simulink model "LV_grid"  (R2021b)
settings: Solver=VariableStepAuto  StartTime=0  StopTime=5.0005  FixedStep=5e-4  RelTol=1e-3
model workspace (MAT data in the model file):
  P2_1 = 3450
  idx = 1
  time_counter = 1
libraries: spsGroundLib x97, spsStairGeneratorLib x96, spsPiSectionLineLib x90, spsThreePhasePISectionLineLib x90, spsVariableInductorLib x48, spsVariableResistorLib x48, spsRMSLib x36, spsThreePhaseVIMeasurementLib x34, spsACVoltageSourceLib x5, spsLinearTransformerLib x5, spsPower3phInstantaneousLib x1, spsThreePhaseMutualInductanceZ1Z0Lib x1
(part 6 of 6)

== system LV_grid/L8/L1 ==
  Pi Section Line : spsPiSectionLineLib/Pi Section Line  LConnTagsString=__new0  RConnTagsString=__new0  Phases=1  PiSections=1  Length=0.0025  Frequency=50  Resistance=0.274  Inductance=0.073  Capacitance=12.74e-9  Measurements=None  Measurements2=None
      settings: SourceProductBaseCode=PS
  Three-Phase PI Section Line : spsThreePhasePISectionLineLib/Three-Phase PI Section Line  LConnTagsString=a|b|c  RConnTagsString=A|B|C  Length=0.0025  Frequency=50  Resistances=[ 0.274 0.959]  Inductances=[ 0.073 0.079]  Capacitances=[12.74e-9 7.751e-9]
  A : PMIOPort  Side=Left
  B : PMIOPort  Port=2  Side=Left
  C : PMIOPort  Port=3  Side=Left
  N : PMIOPort  Port=4  Side=Left
  a : PMIOPort  Port=5  Side=Right
  b : PMIOPort  Port=6  Side=Right
  c : PMIOPort  Port=7  Side=Right
  n : PMIOPort  Port=8  Side=Right
  connections:
  Pi Section Line/LConn1 -- N/RConn1
  Pi Section Line/RConn1 -- n/RConn1
  C/RConn1 -- Three-Phase PI Section Line/LConn3
  B/RConn1 -- Three-Phase PI Section Line/LConn2
  A/RConn1 -- Three-Phase PI Section Line/LConn1
  Three-Phase PI Section Line/RConn3 -- c/RConn1
  Three-Phase PI Section Line/RConn2 -- b/RConn1
  Three-Phase PI Section Line/RConn1 -- a/RConn1

== system LV_grid/L8/L2 ==
  Pi Section Line : spsPiSectionLineLib/Pi Section Line  LConnTagsString=__new0  RConnTagsString=__new0  Phases=1  PiSections=1  Length=0.0025  Frequency=50  Resistance=0.274  Inductance=0.073  Capacitance=12.74e-9  Measurements=None  Measurements2=None
      settings: SourceProductBaseCode=PS
  Three-Phase PI Section Line : spsThreePhasePISectionLineLib/Three-Phase PI Section Line  LConnTagsString=a|b|c  RConnTagsString=A|B|C  Length=0.0025  Frequency=50  Resistances=[ 0.274 0.959]  Inductances=[ 0.073 0.079]  Capacitances=[12.74e-9 7.751e-9]
  A : PMIOPort  Side=Left
  B : PMIOPort  Port=2  Side=Left
  C : PMIOPort  Port=3  Side=Left
  N : PMIOPort  Port=4  Side=Left
  a : PMIOPort  Port=5  Side=Right
  b : PMIOPort  Port=6  Side=Right
  c : PMIOPort  Port=7  Side=Right
  n : PMIOPort  Port=8  Side=Right
  connections:
  Pi Section Line/LConn1 -- N/RConn1
  Pi Section Line/RConn1 -- n/RConn1
  C/RConn1 -- Three-Phase PI Section Line/LConn3
  B/RConn1 -- Three-Phase PI Section Line/LConn2
  A/RConn1 -- Three-Phase PI Section Line/LConn1
  Three-Phase PI Section Line/RConn3 -- c/RConn1
  Three-Phase PI Section Line/RConn2 -- b/RConn1
  Three-Phase PI Section Line/RConn1 -- a/RConn1

== system LV_grid/L8/L3 ==
  Pi Section Line : spsPiSectionLineLib/Pi Section Line  LConnTagsString=__new0  RConnTagsString=__new0  Phases=1  PiSections=1  Length=0.0025  Frequency=50  Resistance=0.274  Inductance=0.073  Capacitance=12.74e-9  Measurements=None  Measurements2=None
      settings: SourceProductBaseCode=PS
  Three-Phase PI Section Line : spsThreePhasePISectionLineLib/Three-Phase PI Section Line  LConnTagsString=a|b|c  RConnTagsString=A|B|C  Length=0.0025  Frequency=50  Resistances=[ 0.274 0.959]  Inductances=[ 0.073 0.079]  Capacitances=[12.74e-9 7.751e-9]
  A : PMIOPort  Side=Left
  B : PMIOPort  Port=2  Side=Left
  C : PMIOPort  Port=3  Side=Left
  N : PMIOPort  Port=4  Side=Left
  a : PMIOPort  Port=5  Side=Right
  b : PMIOPort  Port=6  Side=Right
  c : PMIOPort  Port=7  Side=Right
  n : PMIOPort  Port=8  Side=Right
  connections:
  Pi Section Line/LConn1 -- N/RConn1
  Pi Section Line/RConn1 -- n/RConn1
  C/RConn1 -- Three-Phase PI Section Line/LConn3
  B/RConn1 -- Three-Phase PI Section Line/LConn2
  A/RConn1 -- Three-Phase PI Section Line/LConn1
  Three-Phase PI Section Line/RConn3 -- c/RConn1
  Three-Phase PI Section Line/RConn2 -- b/RConn1
  Three-Phase PI Section Line/RConn1 -- a/RConn1

== system LV_grid/L9/L1 ==
  Pi Section Line : spsPiSectionLineLib/Pi Section Line  LConnTagsString=__new0  RConnTagsString=__new0  Phases=1  PiSections=1  Length=0.0025  Frequency=50  Resistance=0.274  Inductance=0.073  Capacitance=12.74e-9  Measurements=None  Measurements2=None
      settings: SourceProductBaseCode=PS
  Three-Phase PI Section Line : spsThreePhasePISectionLineLib/Three-Phase PI Section Line  LConnTagsString=a|b|c  RConnTagsString=A|B|C  Length=0.0025  Frequency=50  Resistances=[ 0.274 0.959]  Inductances=[ 0.073 0.079]  Capacitances=[12.74e-9 7.751e-9]
  A : PMIOPort  Side=Left
  B : PMIOPort  Port=2  Side=Left
  C : PMIOPort  Port=3  Side=Left
  N : PMIOPort  Port=4  Side=Left
  a : PMIOPort  Port=5  Side=Right
  b : PMIOPort  Port=6  Side=Right
  c : PMIOPort  Port=7  Side=Right
  n : PMIOPort  Port=8  Side=Right
  connections:
  Pi Section Line/LConn1 -- N/RConn1
  Pi Section Line/RConn1 -- n/RConn1
  C/RConn1 -- Three-Phase PI Section Line/LConn3
  B/RConn1 -- Three-Phase PI Section Line/LConn2
  A/RConn1 -- Three-Phase PI Section Line/LConn1
  Three-Phase PI Section Line/RConn3 -- c/RConn1
  Three-Phase PI Section Line/RConn2 -- b/RConn1
  Three-Phase PI Section Line/RConn1 -- a/RConn1

== system LV_grid/L9/L2 ==
  Pi Section Line : spsPiSectionLineLib/Pi Section Line  LConnTagsString=__new0  RConnTagsString=__new0  Phases=1  PiSections=1  Length=0.0025  Frequency=50  Resistance=0.274  Inductance=0.073  Capacitance=12.74e-9  Measurements=None  Measurements2=None
      settings: SourceProductBaseCode=PS
  Three-Phase PI Section Line : spsThreePhasePISectionLineLib/Three-Phase PI Section Line  LConnTagsString=a|b|c  RConnTagsString=A|B|C  Length=0.0025  Frequency=50  Resistances=[ 0.274 0.959]  Inductances=[ 0.073 0.079]  Capacitances=[12.74e-9 7.751e-9]
  A : PMIOPort  Side=Left
  B : PMIOPort  Port=2  Side=Left
  C : PMIOPort  Port=3  Side=Left
  N : PMIOPort  Port=4  Side=Left
  a : PMIOPort  Port=5  Side=Right
  b : PMIOPort  Port=6  Side=Right
  c : PMIOPort  Port=7  Side=Right
  n : PMIOPort  Port=8  Side=Right
  connections:
  Pi Section Line/LConn1 -- N/RConn1
  Pi Section Line/RConn1 -- n/RConn1
  C/RConn1 -- Three-Phase PI Section Line/LConn3
  B/RConn1 -- Three-Phase PI Section Line/LConn2
  A/RConn1 -- Three-Phase PI Section Line/LConn1
  Three-Phase PI Section Line/RConn3 -- c/RConn1
  Three-Phase PI Section Line/RConn2 -- b/RConn1
  Three-Phase PI Section Line/RConn1 -- a/RConn1

== system LV_grid/L9/L3 ==
  Pi Section Line : spsPiSectionLineLib/Pi Section Line  LConnTagsString=__new0  RConnTagsString=__new0  Phases=1  PiSections=1  Length=0.0025  Frequency=50  Resistance=0.274  Inductance=0.073  Capacitance=12.74e-9  Measurements=None  Measurements2=None
      settings: SourceProductBaseCode=PS
  Three-Phase PI Section Line : spsThreePhasePISectionLineLib/Three-Phase PI Section Line  LConnTagsString=a|b|c  RConnTagsString=A|B|C  Length=0.0025  Frequency=50  Resistances=[ 0.274 0.959]  Inductances=[ 0.073 0.079]  Capacitances=[12.74e-9 7.751e-9]
  A : PMIOPort  Side=Left
  B : PMIOPort  Port=2  Side=Left
  C : PMIOPort  Port=3  Side=Left
  N : PMIOPort  Port=4  Side=Left
  a : PMIOPort  Port=5  Side=Right
  b : PMIOPort  Port=6  Side=Right
  c : PMIOPort  Port=7  Side=Right
  n : PMIOPort  Port=8  Side=Right
  connections:
  Pi Section Line/LConn1 -- N/RConn1
  Pi Section Line/RConn1 -- n/RConn1
  C/RConn1 -- Three-Phase PI Section Line/LConn3
  B/RConn1 -- Three-Phase PI Section Line/LConn2
  A/RConn1 -- Three-Phase PI Section Line/LConn1
  Three-Phase PI Section Line/RConn3 -- c/RConn1
  Three-Phase PI Section Line/RConn2 -- b/RConn1
  Three-Phase PI Section Line/RConn1 -- a/RConn1

== system LV_grid/L9/L4 ==
  Pi Section Line : spsPiSectionLineLib/Pi Section Line  LConnTagsString=__new0  RConnTagsString=__new0  Phases=1  PiSections=1  Length=0.0025  Frequency=50  Resistance=0.274  Inductance=0.073  Capacitance=12.74e-9  Measurements=None  Measurements2=None
      settings: SourceProductBaseCode=PS
  Three-Phase PI Section Line : spsThreePhasePISectionLineLib/Three-Phase PI Section Line  LConnTagsString=a|b|c  RConnTagsString=A|B|C  Length=0.0025  Frequency=50  Resistances=[ 0.274 0.959]  Inductances=[ 0.073 0.079]  Capacitances=[12.74e-9 7.751e-9]
  A : PMIOPort  Side=Left
  B : PMIOPort  Port=2  Side=Left
  C : PMIOPort  Port=3  Side=Left
  N : PMIOPort  Port=4  Side=Left
  a : PMIOPort  Port=5  Side=Right
  b : PMIOPort  Port=6  Side=Right
  c : PMIOPort  Port=7  Side=Right
  n : PMIOPort  Port=8  Side=Right
  connections:
  Pi Section Line/LConn1 -- N/RConn1
  Pi Section Line/RConn1 -- n/RConn1
  C/RConn1 -- Three-Phase PI Section Line/LConn3
  B/RConn1 -- Three-Phase PI Section Line/LConn2
  A/RConn1 -- Three-Phase PI Section Line/LConn1
  Three-Phase PI Section Line/RConn3 -- c/RConn1
  Three-Phase PI Section Line/RConn2 -- b/RConn1
  Three-Phase PI Section Line/RConn1 -- a/RConn1

== system LV_grid/L9/L5 ==
  Pi Section Line : spsPiSectionLineLib/Pi Section Line  LConnTagsString=__new0  RConnTagsString=__new0  Phases=1  PiSections=1  Length=0.0025  Frequency=50  Resistance=0.274  Inductance=0.073  Capacitance=12.74e-9  Measurements=None  Measurements2=None
      settings: SourceProductBaseCode=PS
  Three-Phase PI Section Line : spsThreePhasePISectionLineLib/Three-Phase PI Section Line  LConnTagsString=a|b|c  RConnTagsString=A|B|C  Length=0.0025  Frequency=50  Resistances=[ 0.274 0.959]  Inductances=[ 0.073 0.079]  Capacitances=[12.74e-9 7.751e-9]
  A : PMIOPort  Side=Left
  B : PMIOPort  Port=2  Side=Left
  C : PMIOPort  Port=3  Side=Left
  N : PMIOPort  Port=4  Side=Left
  a : PMIOPort  Port=5  Side=Right
  b : PMIOPort  Port=6  Side=Right
  c : PMIOPort  Port=7  Side=Right
  n : PMIOPort  Port=8  Side=Right
  connections:
  Pi Section Line/LConn1 -- N/RConn1
  Pi Section Line/RConn1 -- n/RConn1
  C/RConn1 -- Three-Phase PI Section Line/LConn3
  B/RConn1 -- Three-Phase PI Section Line/LConn2
  A/RConn1 -- Three-Phase PI Section Line/LConn1
  Three-Phase PI Section Line/RConn3 -- c/RConn1
  Three-Phase PI Section Line/RConn2 -- b/RConn1
  Three-Phase PI Section Line/RConn1 -- a/RConn1

== matlab function LV_grid/B13/MATLAB Function ==
  data: u input; y output
function y = Gaussian(u)
mean = 0;
sigma = 1e-4;

y = u + mean + sigma.*randn(size(u));

== matlab function LV_grid/B16/MATLAB Function ==
  data: u input; y output
function y = Gaussian(u)
mean = 0;
sigma = 1e-4;

y = u + mean + sigma.*randn(size(u));

== matlab function LV_grid/B17/MATLAB Function ==
  data: u input; y output
function y = Gaussian(u)
mean = 0;
sigma = 1e-4;

y = u + mean + sigma.*randn(size(u));

== matlab function LV_grid/B18/MATLAB Function ==
  data: u input; y output
function y = Gaussian(u)
mean = 0;
sigma = 1e-4;

y = u + mean + sigma.*randn(size(u));

== matlab function LV_grid/B19/MATLAB Function ==
  data: u input; y output
function y = Gaussian(u)
mean = 0;
sigma = 1e-4;

y = u + mean + sigma.*randn(size(u));

== matlab function LV_grid/B1/MATLAB Function ==
  data: u input; y output
function y = Gaussian(u)
mean = 0;
sigma = 1e-4;

y = u + mean + sigma.*randn(size(u));

== matlab function LV_grid/B20/MATLAB Function ==
  data: u input; y output
function y = Gaussian(u)
mean = 0;
sigma = 1e-4;

y = u + mean + sigma.*randn(size(u));

== matlab function LV_grid/B21/MATLAB Function ==
  data: u input; y output
function y = Gaussian(u)
mean = 0;
sigma = 1e-4;

y = u + mean + sigma.*randn(size(u));

== matlab function LV_grid/B24/MATLAB Function ==
  data: u input; y output
function y = Gaussian(u)
mean = 0;
sigma = 1e-4;

y = u + mean + sigma.*randn(size(u));

== matlab function LV_grid/B25/MATLAB Function ==
  data: u input; y output
function y = Gaussian(u)
mean = 0;
sigma = 1e-4;

y = u + mean + sigma.*randn(size(u));

== matlab function LV_grid/B26/MATLAB Function ==
  data: u input; y output
function y = Gaussian(u)
mean = 0;
sigma = 1e-4;

y = u + mean + sigma.*randn(size(u));

== matlab function LV_grid/B27/MATLAB Function ==
  data: u input; y output
function y = Gaussian(u)
mean = 0;
sigma = 1e-4;

y = u + mean + sigma.*randn(size(u));

== matlab function LV_grid/B29/MATLAB Function ==
  data: u input; y output
function y = Gaussian(u)
mean = 0;
sigma = 1e-4;

y = u + mean + sigma.*randn(size(u));

== matlab function LV_grid/B30/MATLAB Function ==
  data: u input; y output
function y = Gaussian(u)
mean = 0;
sigma = 1e-4;

y = u + mean + sigma.*randn(size(u));

== matlab function LV_grid/B31/MATLAB Function ==
  data: u input; y output
function y = Gaussian(u)
mean = 0;
sigma = 1e-4;

y = u + mean + sigma.*randn(size(u));

== matlab function LV_grid/B33/MATLAB Function ==
  data: u input; y output
function y = Gaussian(u)
mean = 0;
sigma = 1e-4;

y = u + mean + sigma.*randn(size(u));

== matlab function LV_grid/B2/MATLAB Function1 ==
  data: u input; y output
function y = Gaussian(u)
mean = 0;
sigma = 1e-4;

y = u + mean + sigma.*randn(size(u));

== matlab function LV_grid/B8/MATLAB Function ==
  data: u input; y output
function y = Gaussian(u)
mean = 0;
sigma = 1e-4;

y = u + mean + sigma.*randn(size(u));

== matlab function LV_grid/B14/MATLAB Function ==
  data: u input; y output
function y = Gaussian(u)
mean = 0;
sigma = 1e-4;

y = u + mean + sigma.*randn(size(u));

== matlab function LV_grid/B15/MATLAB Function ==
  data: u input; y output
function y = Gaussian(u)
mean = 0;
sigma = 1e-4;

y = u + mean + sigma.*randn(size(u));

== matlab function LV_grid/B22/MATLAB Function ==
  data: u input; y output
function y = Gaussian(u)
mean = 0;
sigma = 1e-4;

y = u + mean + sigma.*randn(size(u));

== matlab function LV_grid/B23/MATLAB Function ==
  data: u input; y output
function y = Gaussian(u)
mean = 0;
sigma = 1e-4;

y = u + mean + sigma.*randn(size(u));

== matlab function LV_grid/B28/MATLAB Function ==
  data: u input; y output
function y = Gaussian(u)
mean = 0;
sigma = 1e-4;

y = u + mean + sigma.*randn(size(u));

== matlab function LV_grid/B32/MATLAB Function ==
  data: u input; y output
function y = Gaussian(u)
mean = 0;
sigma = 1e-4;

y = u + mean + sigma.*randn(size(u));

== matlab function LV_grid/B3/MATLAB Function ==
  data: u input; y output
function y = Gaussian(u)
mean = 0;
sigma = 1e-4;

y = u + mean + sigma.*randn(size(u));

== matlab function LV_grid/B3/MATLAB Function1 ==
  data: u input; y output
function y = Gaussian(u)
mean = 0;
sigma = 1e-4;

y = u + mean + sigma.*randn(size(u));

== matlab function LV_grid/B4/MATLAB Function ==
  data: u input; y output
function y = Gaussian(u)
mean = 0;
sigma = 1e-4;

y = u + mean + sigma.*randn(size(u));

== matlab function LV_grid/B4/MATLAB Function1 ==
  data: u input; y output
function y = Gaussian(u)
mean = 0;
sigma = 1e-4;

y = u + mean + sigma.*randn(size(u));

== matlab function LV_grid/B5/MATLAB Function ==
  data: u input; y output
function y = Gaussian(u)
mean = 0;
sigma = 1e-4;

y = u + mean + sigma.*randn(size(u));

== matlab function LV_grid/B6/MATLAB Function ==
  data: u input; y output
function y = Gaussian(u)
mean = 0;
sigma = 1e-4;

y = u + mean + sigma.*randn(size(u));

== matlab function LV_grid/B2/MATLAB Function ==
  data: u input; y output
function y = Gaussian(u)
mean = 0;
sigma = 1e-4;

y = u + mean + sigma.*randn(size(u));

== matlab function LV_grid/B7/MATLAB Function ==
  data: u input; y output
function y = Gaussian(u)
mean = 0;
sigma = 1e-4;

y = u + mean + sigma.*randn(size(u));

== matlab function LV_grid/B9/MATLAB Function ==
  data: u input; y output
function y = Gaussian(u)
mean = 0;
sigma = 1e-4;

y = u + mean + sigma.*randn(size(u));

== matlab function LV_grid/B10/MATLAB Function ==
  data: u input; y output
function y = Gaussian(u)
mean = 0;
sigma = 1e-4;

y = u + mean + sigma.*randn(size(u));

== matlab function LV_grid/B11/MATLAB Function ==
  data: u input; y output
function y = Gaussian(u)
mean = 0;
sigma = 1e-4;

y = u + mean + sigma.*randn(size(u));

== matlab function LV_grid/B12/MATLAB Function ==
  data: u input; y output
function y = Gaussian(u)
mean = 0;
sigma = 1e-4;

y = u + mean + sigma.*randn(size(u));
